simulink model "Option1"  (R2023b)
settings: Solver=ode4  StartTime=0.0  StopTime=25  FixedStep=dT  RelTol=1e-3
undefined symbols (not defined in the file): a, B1, B2, J1, J2, K
settings Model: Creator=oscar  LastModifiedBy=huert

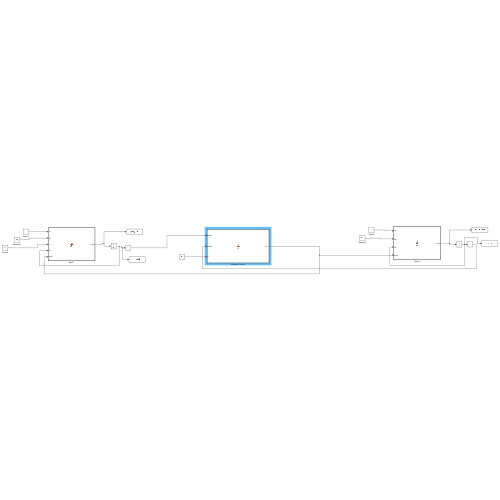
[thumbnail: Simulink's stored preview of the top-level diagram]
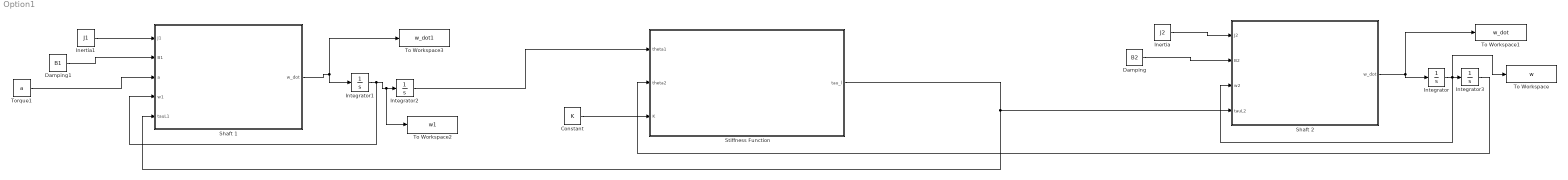
== system Option1 ==
  Constant : Constant  Value=K
  Damping : Constant  Value=B2
  Damping1 : Constant  Value=B1
  Inertia : Constant  Value=J2
  Inertia1 : Constant  Value=J1
  Integrator : Integrator  UpperSaturationLimit=1000
  Integrator1 : Integrator  UpperSaturationLimit=1000
  Integrator2 : Integrator
  Integrator3 : Integrator
  Shaft 1 : MATLAB Function  TreatAsAtomicUnit=on
  Shaft 2 : MATLAB Function  TreatAsAtomicUnit=on
  Stiffness Function : MATLAB Function  TreatAsAtomicUnit=on
  To Workspace : ToWorkspace  VariableName=w  SaveFormat=Structure With Time  SampleTime=-1
  To Workspace1 : ToWorkspace  VariableName=w_dot  SaveFormat=Structure With Time  SampleTime=-1
  To Workspace2 : ToWorkspace  VariableName=w1  SaveFormat=Structure With Time  SampleTime=-1
  To Workspace3 : ToWorkspace  VariableName=w_dot1  SaveFormat=Structure With Time  SampleTime=-1
  Torque1 : Constant  Value=a
  wires:
  Shaft 2/1(w_dot) -> To Workspace1/1, Integrator/1
  Inertia/1 -> Shaft 2/1(J2)
  Damping/1 -> Shaft 2/2(B2)
  Integrator/1 -> To Workspace/1, Integrator3/1, Shaft 2/3(w2)
  Torque1/1 -> Shaft 1/3(a)
  Damping1/1 -> Shaft 1/2(B1)
  Inertia1/1 -> Shaft 1/1(J1)
  Shaft 1/1(w_dot) -> To Workspace3/1, Integrator1/1
  Stiffness Function/1(tau_l) -> Shaft 2/4(tauL2), Shaft 1/5(tauL1)
  Integrator1/1 -> Shaft 1/4(w1), To Workspace2/1, Integrator2/1
  Integrator2/1 -> Stiffness Function/1(theta1)
  Constant/1 -> Stiffness Function/3(K)
  Integrator3/1 -> Stiffness Function/2(theta2)

== matlab function Option1/Shaft 1 ==
  data: J1 input; w_dot output; B1 input; a input; w1 input; tauL1 input
function w_dot = fcn(J1, B1, a, w1, tauL1)

w_dot = (1/J1)*(a - tauL1 - (B1*w1));

end

== matlab function Option1/Shaft 2 ==
  data: J2 input; w_dot output; B2 input; w2 input; tauL2 input
function w_dot = fcn(J2, B2, w2, tauL2)

w_dot = (1/J2)*(tauL2 - (B2*w2));

end

== matlab function Option1/Stiffness Function ==
  data: theta1 input; tau_l output; theta2 input; K input
function tau_l = fcn(theta1, theta2, K)

tau_l = K*(theta1 - theta2);
    
end
